simulink model "SH_control"  (R2023b)
settings: configuration reference "ctrl_tsk_conf" (kept outside this file)
settings Model: DataDictionary=fmuGenerationDictionay.sldd  Creator=Veimar  LastModifiedBy=Veimar
settings ConfigSetRef: SourceName=ctrl_tsk_conf

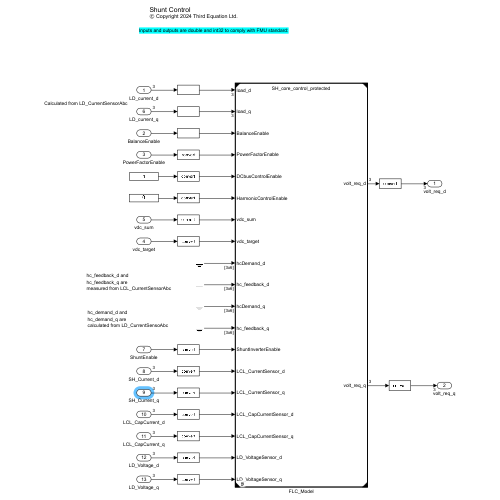
[thumbnail: Simulink's stored preview of the top-level diagram]
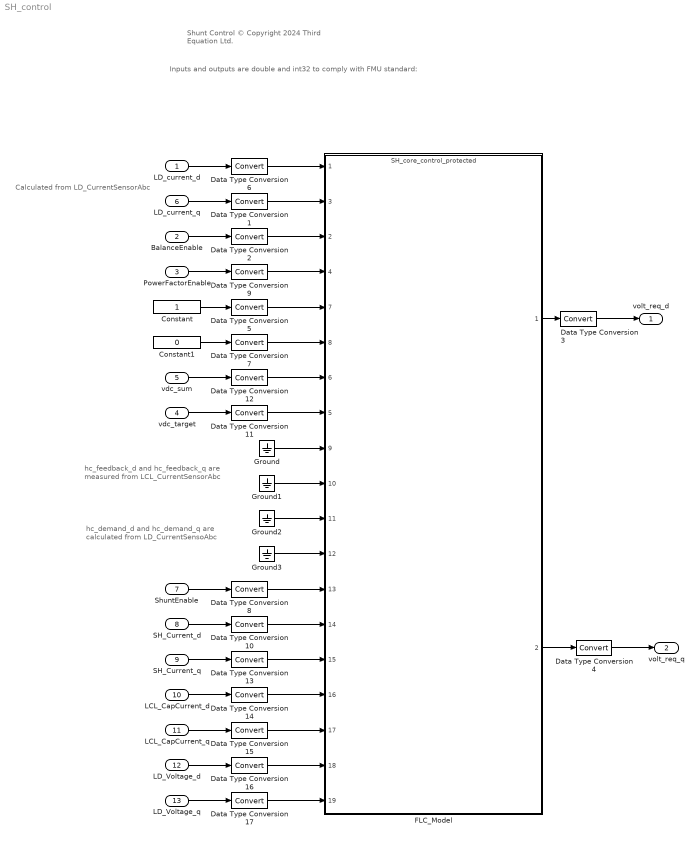
== system SH_control ==
  note: Calculated from LD_CurrentSensorAbc
  note: Shunt Control
      | © Copyright 2024 Third Equation Ltd.
  note: Inputs and outputs are double and int32 to comply with FMU standard:
  note: hc_demand_d and
      | hc_demand_q are
      | calculated from LD_CurrentSensoAbc
  note: hc_feedback_d and
      | hc_feedback_q are
      | measured from LCL_CurrentSensorAbc
  LD_current_d : Inport  OutDataTypeStr=double  PortDimensions=3
  BalanceEnable : Inport  Port=2  OutDataTypeStr=int32  PortDimensions=1
  PowerFactorEnable : Inport  Port=3  OutDataTypeStr=int32  PortDimensions=1
  vdc_target : Inport  Port=4  OutDataTypeStr=double  PortDimensions=1
  vdc_sum : Inport  Port=5  OutDataTypeStr=double  PortDimensions=1
  LD_current_q : Inport  Port=6  OutDataTypeStr=double  PortDimensions=3
  ShuntEnable : Inport  Port=7  OutDataTypeStr=int32  PortDimensions=1
  SH_Current_d : Inport  Port=8  OutDataTypeStr=double  PortDimensions=3
  SH_Current_q : Inport  Port=9  OutDataTypeStr=double  PortDimensions=3
  LCL_CapCurrent_d : Inport  Port=10  OutDataTypeStr=double  PortDimensions=3
  LCL_CapCurrent_q : Inport  Port=11  OutDataTypeStr=double  PortDimensions=3
  LD_Voltage_d : Inport  Port=12  OutDataTypeStr=double  PortDimensions=3
  LD_Voltage_q : Inport  Port=13  OutDataTypeStr=double  PortDimensions=3
  Constant : Constant  OutDataTypeStr=int32
  Constant1 : Constant  Value=0  OutDataTypeStr=int32
  Data Type Conversion{1..17} (17 alike) : DataTypeConversion  SaturateOnIntegerOverflow=off  RndMeth=Floor
  FLC_Model : ModelReference  ModelNameDialog=SH_core_control_protected.slxp  ModelReferenceVersion=1.55  CopyOfModelProtected=on
      settings: PortSchema="{\"entries\":[{\"content\":{\"sides\":[{\"content\":{\"connectorIds\":[\"In1\",\"In3\",\"In2\",\"In4\",\"In7\",\"In8\",\"In6\",\"In5\",\"In9\",\"In10\",\"In11\",\"In12\",\"In13\",\"In14\",\"In15\",\"In16\",\"In17\",\"In18\",\"In19\"]},\"type\":\"ConnectorPlacement.EquallySpacedRectSide\",\"uuid\":\"23c75067-9470-41eb-93ec-30ae2c10cb0d\"},{\"content\":{\"connectorIds\":[\"Out1\",\"Out2\"],\"side\":\"RIGHT\"},\"type\":\"ConnectorPlacement.EquallySpacedRectSide\",\"uuid\":\"e9e1d1ef-f621-4d5e-b012-882bc6e1d937\"},{\"content\":{\"side\":\"TOP\"},\"type\":\"ConnectorPlacement.EquallySpacedRectSide\",\"uuid\":\"2453977c-ee77-410e-a5e8-00be7c4d652d\"}]},\"type\":\"ConnectorPlacement.EquallySpacedConnector\",\"uuid\":\"3c4f9718-bd97-403d-90d5-b0be8a0f7b23\"}],\"packageUris\":[\"http://schema.mathworks.com/mf0/Connector/R2020b\"],\"version\":\"1.0\"}"
  Ground{,1..3} (4 alike) : Ground
  volt_req_d : Outport  OutDataTypeStr=double  PortDimensions=3
  volt_req_q : Outport  Port=2  OutDataTypeStr=double  PortDimensions=3
  wires:
  LD_current_d/1 -> Data Type Conversion6/1
  Data Type Conversion6/1 -> FLC_Model/1
  BalanceEnable/1 -> Data Type Conversion2/1
  FLC_Model/1 -> Data Type Conversion3/1
  Data Type Conversion3/1 -> volt_req_d/1
  Data Type Conversion4/1 -> volt_req_q/1
  PowerFactorEnable/1 -> Data Type Conversion9/1
  FLC_Model/2 -> Data Type Conversion4/1
  vdc_target/1 -> Data Type Conversion11/1
  Data Type Conversion11/1 -> FLC_Model/5
  vdc_sum/1 -> Data Type Conversion12/1
  Data Type Conversion12/1 -> FLC_Model/6
  Constant/1 -> Data Type Conversion5/1
  Data Type Conversion9/1 -> FLC_Model/4
  Constant1/1 -> Data Type Conversion7/1
  Data Type Conversion2/1 -> FLC_Model/2
  Ground/1 -> FLC_Model/9
  Ground1/1 -> FLC_Model/10
  Ground2/1 -> FLC_Model/11
  Ground3/1 -> FLC_Model/12
  Data Type Conversion1/1 -> FLC_Model/3
  LD_current_q/1 -> Data Type Conversion1/1
  Data Type Conversion5/1 -> FLC_Model/7
  Data Type Conversion7/1 -> FLC_Model/8
  ShuntEnable/1 -> Data Type Conversion8/1
  Data Type Conversion8/1 -> FLC_Model/13
  Data Type Conversion10/1 -> FLC_Model/14
  SH_Current_d/1 -> Data Type Conversion10/1
  SH_Current_q/1 -> Data Type Conversion13/1
  Data Type Conversion13/1 -> FLC_Model/15
  LCL_CapCurrent_d/1 -> Data Type Conversion14/1
  LCL_CapCurrent_q/1 -> Data Type Conversion15/1
  Data Type Conversion14/1 -> FLC_Model/16
  Data Type Conversion15/1 -> FLC_Model/17
  LD_Voltage_d/1 -> Data Type Conversion16/1
  LD_Voltage_q/1 -> Data Type Conversion17/1
  Data Type Conversion16/1 -> FLC_Model/18
  Data Type Conversion17/1 -> FLC_Model/19
